simulink model "passive_suspension"  (R2025a)
settings: Solver=ode23s  StartTime=0.0  StopTime=T_sim  RelTol=1e-3
undefined symbols (not defined in the file): cs, ks, kt, ms, mus, zs_static, zus_static
settings Model: Creator=Anderson  LastModifiedBy=Anderson
settings DataIOCC: SaveFormat=Array

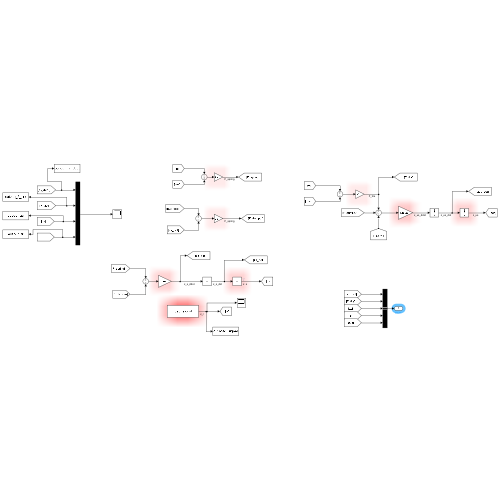
[thumbnail: Simulink's stored preview of the top-level diagram]
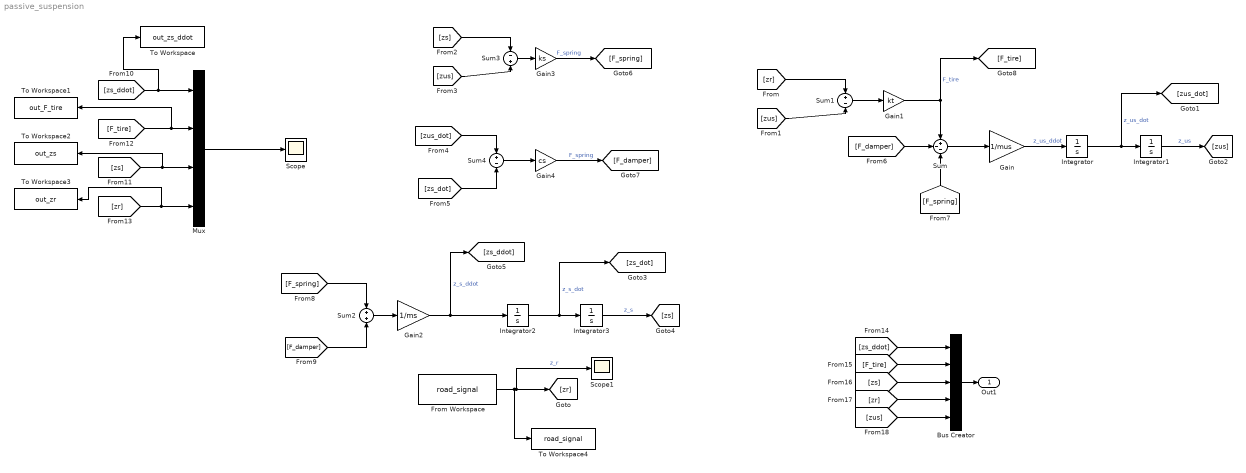
== system passive_suspension ==
  Bus Creator : BusCreator  Inputs=5
  From Workspace : FromWorkspace  VariableName=road_signal
  Gain : Gain  Gain=1/mus
  Gain1 : Gain  Gain=kt
  Gain2 : Gain  Gain=1/ms
  Gain3 : Gain  Gain=ks
  Gain4 : Gain  Gain=cs
  Integrator : Integrator
  Integrator1 : Integrator  InitialCondition=zus_static
  Integrator2 : Integrator
  Integrator3 : Integrator  InitialCondition=zs_static
  Mux : Mux
  Scope : Scope
      settings: ActiveDisplayYMinimum=-6868.1819363859859  ActiveDisplayYMaximum=4567.23132626511
  Scope1 : Scope
      settings: ActiveDisplayYMinimum=-0.015059257121935982  ActiveDisplayYMaximum=0.11687885581387557
  Sum : Sum  Inputs=+--
  Sum1 : Sum  Inputs=+-
  Sum2 : Sum
  Sum3 : Sum  Inputs=-+
  Sum4 : Sum  Inputs=+-
  To Workspace : ToWorkspace  VariableName=out_zs_ddot  SampleTime=-1
  To Workspace1 : ToWorkspace  VariableName=out_F_tire  SampleTime=-1
  To Workspace2 : ToWorkspace  VariableName=out_zs  SampleTime=-1
  To Workspace3 : ToWorkspace  VariableName=out_zr  SampleTime=-1
  To Workspace4 : ToWorkspace  VariableName=road_signal  SaveFormat=Timeseries  SampleTime=-1
  Out1 : Outport
  wires:
  From Workspace/1 -> [zr], Scope1/1, To Workspace4/1  "z_r"
  Integrator/1 -> [zus_dot], Integrator1/1  "z_us_dot"
  Gain/1 -> Integrator/1  "z_us_ddot​"
  Integrator1/1 -> [zus]  "z_us"
  Sum/1 -> Gain/1
  [zr] -> Sum1/1
  [zus] -> Sum1/2
  Sum1/1 -> Gain1/1
  Gain1/1 -> Sum/1, [F_tire]  "F_tire"
  Gain2/1 -> [zs_ddot], Integrator2/1  "z_s_ddot"
  Integrator2/1 -> [zs_dot], Integrator3/1  "z_s_dot"
  Integrator3/1 -> [zs]  "z_s"
  Sum2/1 -> Gain2/1
  [zs] -> Sum3/1
  [zus] -> Sum3/2
  Sum3/1 -> Gain3/1
  Gain3/1 -> [F_spring]  "F_spring"
  [zus_dot] -> Sum4/1
  [zs_dot] -> Sum4/2
  Sum4/1 -> Gain4/1
  Gain4/1 -> [F_damper]  "F_spring"
  [F_spring] -> Sum/3
  [F_damper] -> Sum/2
  [F_spring] -> Sum2/1
  [F_damper] -> Sum2/2
  [zs_ddot] -> To Workspace/1, Mux/1
  [F_tire] -> To Workspace1/1, Mux/2
  [zs] -> To Workspace2/1, Mux/3
  [zr] -> To Workspace3/1, Mux/4
  Mux/1 -> Scope/1
  [zus] -> Bus Creator/5
  [zr] -> Bus Creator/4
  [zs] -> Bus Creator/3
  [F_tire] -> Bus Creator/2
  [zs_ddot] -> Bus Creator/1
  Bus Creator/1 -> Out1/1
